simulink model "Ex_1"  (R2019a)
settings: Solver=VariableStepAuto  StartTime=0.0  StopTime=10.0  RelTol=1e-3
libraries: cstblocks x2, simulink x1
settings Model: Creator=sselvaraja2018  LastModifiedBy=sselvaraja2018

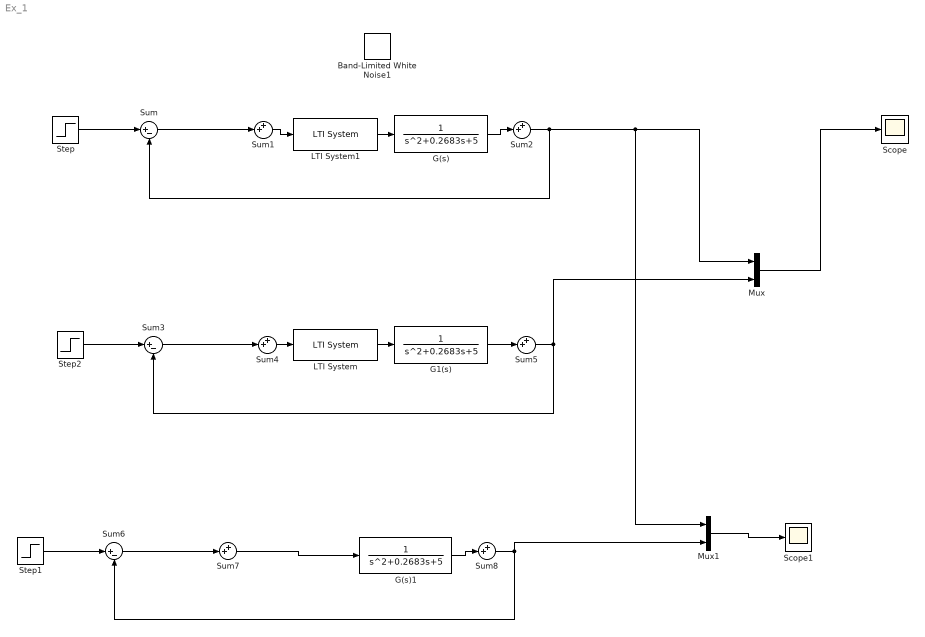
== system Ex_1 ==
  Band-Limited White Noise1 : simulink/Sources/Band-Limited White Noise  Cov=[0.00000001]  Ts=0.001  seed=[23341]
  G(s) : TransferFcn  Denominator=[1 0.2683 5]
  G(s)1 : TransferFcn  Denominator=[1 0.2683 5]
  G1(s) : TransferFcn  Denominator=[1 0.2683 5]
  LTI System : cstblocks/LTI System  sys=K2  IC=[]
  LTI System1 : cstblocks/LTI System  sys=K1  IC=[]
  Mux : Mux  Inputs=2
  Mux1 : Mux  Inputs=2
  Scope : Scope
  Scope1 : Scope
  Step : Step  SampleTime=0
  Step1 : Step  SampleTime=0
  Step2 : Step  SampleTime=0
  Sum : Sum  Inputs=|+-
  Sum{1..2,4..5,7..8} (6 alike) : Sum  Inputs=++|
  Sum3 : Sum  Inputs=|+-
  Sum6 : Sum  Inputs=|+-
  wires:
  ? -> Sum1/1
  Step/1 -> Sum/1
  Sum/1 -> Sum1/2
  G(s)/1 -> Sum2/2
  Sum2/1 -> Mux1/1, Mux/1, Sum/2
  Sum4/1 -> LTI System/1
  Sum3/1 -> Sum4/2
  Step2/1 -> Sum3/1
  Sum5/1 -> Mux/2, Sum3/2
  G1(s)/1 -> Sum5/2
  Mux/1 -> Scope/1
  Sum1/1 -> LTI System1/1
  LTI System1/1 -> G(s)/1
  LTI System/1 -> G1(s)/1
  ? -> Sum4/1
  ? -> Sum5/1
  ? -> Sum2/1
  Sum6/1 -> Sum7/2
  Step1/1 -> Sum6/1
  Sum8/1 -> Mux1/2, Sum6/2
  G(s)1/1 -> Sum8/2
  Sum7/1 -> G(s)1/1
  ? -> Sum8/1
  Mux1/1 -> Scope1/1
